simulink model "Autovessel_medPI"  (R2018a)
settings: Solver=FixedStepAuto  StartTime=0.0  StopTime=inf  RelTol=1e-3  EnableMultiTasking=on
libraries: arduinolib x4, simulink x2
settings Model: SimulationMode=external  ExtModeTrigDuration=2  Creator=Christoffer Lauknes  LastModifiedBy=Christoffer Lauknes
settings OptimizationCC: EnhancedBackFolding=on  PassReuseOutputArgsThreshold=0  MaxStackSize=64  OptimizeBlockOrder=speed  DifferentSizesBufferReuse=on  OptimizationCustomize=off
settings DebuggingCC: ParameterTunabilityLossMsg=error
settings HardwareCC: ProdBitPerInt=16  ProdBitPerPointer=16  ProdBitPerSizeT=16  ProdBitPerPtrDiffT=16  ProdLargestAtomicFloat=None  ProdWordSize=8  ProdHWDeviceType=Atmel->AVR  UseEmbeddedCoderFeatures=off
settings SFSimCC: MATLABDynamicMemAlloc=off
settings RTWCC: SystemTargetFile=ert.tlc  HardwareBoard=Arduino Mega 2560  TLCOptions=-aInlineSetEventsForThisBaseRateFcn=TLC_FALSE -aSuppressMultiTaskScheduler=TLC_FALSE -aRateBasedStepFcn=1  TemplateMakefile=ert_default_tmf  GenerateReport=on  Toolchain=Arduino AVR  BuildConfiguration=Faster Runs  LaunchReport=on
settings CodeAppCC: ForceParamTrailComments=on  OperatorAnnotations=on
settings ERTTargetCC: ERTCustomFileBanners=off  SupportContinuousTime=on  SupportNonInlinedSFcns=on  RemoveResetFunc=off  SupportVariableSizeSignals=on  ModelStepFunctionPrototypeControlCompliant=off

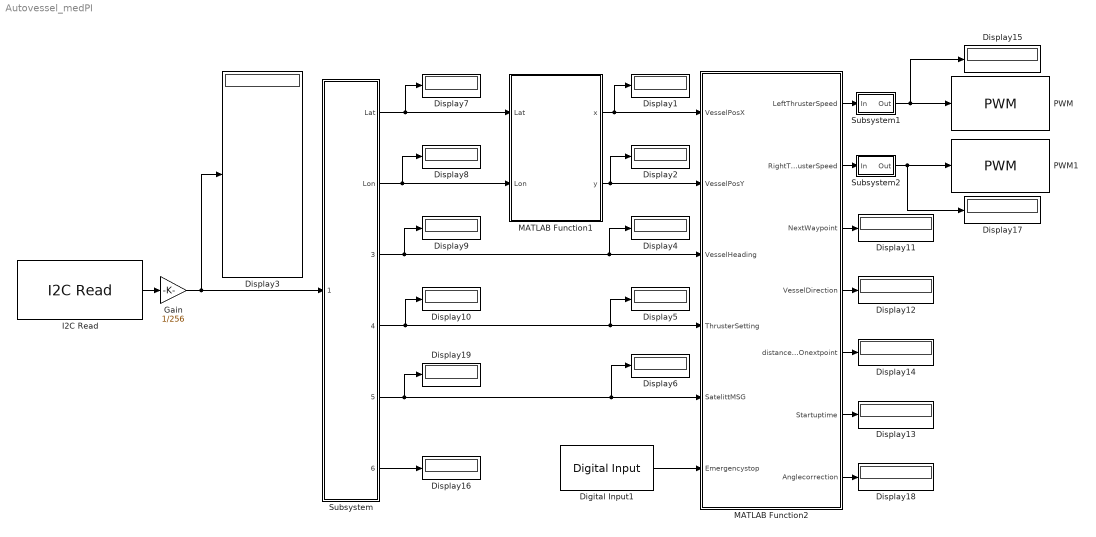
== system Autovessel_medPI ==
  Digital Input1 : arduinolib/Digital Input  pinNumber=30  sampleTime=0.1  blockPlatform=arduino
      settings: SourceProductName=Simulink Support Package for Arduino Hardware
  Display{1..19} (19 alike) : Display
  Gain : Gain  Gain=1/256  OutDataTypeStr=double
  I2C Read : arduinolib/I2C Read  SlaveAddress_=hex2dec( '48' )  RegisterAddressEnable=off  RegisterAddress_=hex2dec( '20' )  Datatype=uint16  ByteOrder=Big Endian  Datalength_=13  SampleTime_=0.1  blockPlatform=arduino
      settings: SourceProductName=Simulink Support Package for Arduino Hardware  SourceProductBaseCode=ARDUINO
  MATLAB Function1 : MATLAB Function  TreatAsAtomicUnit=on
  MATLAB Function2 : MATLAB Function  TreatAsAtomicUnit=on
  PWM : arduinolib/PWM  pinNumber=10  EnableInputFrequency=off  InitialFrequency=2000  InitialDutyCycle=0  NotificationType=None  blockPlatform=arduino
  PWM1 : arduinolib/PWM  pinNumber=12  EnableInputFrequency=off  InitialFrequency=2000  InitialDutyCycle=0  NotificationType=None  blockPlatform=arduino
  Subsystem : Subsystem
  Subsystem1 : Subsystem
  Subsystem2 : Subsystem
  wires:
  MATLAB Function2/1(LeftThrusterSpeed) -> Subsystem1/1(In)
  MATLAB Function2/2(RightThrusterSpeed) -> Subsystem2/1(In)
  MATLAB Function2/3(NextWaypoint) -> Display11/1
  Subsystem/6(Counter) -> Display16/1
  MATLAB Function2/5(distanceTOnextpoint) -> Display14/1
  Subsystem/3(Course) -> Display9/1, Display4/1, MATLAB Function2/3(VesselHeading)
  MATLAB Function2/4(VesselDirection) -> Display12/1
  Subsystem/4(Setting) -> Display10/1, Display5/1, MATLAB Function2/4(ThrusterSetting)
  Subsystem/2(Lon) -> Display8/1, MATLAB Function1/2(Lon)
  Gain/1 -> Display3/1, Subsystem/1(Slavedata)
  MATLAB Function1/1(x) -> Display1/1, MATLAB Function2/1(VesselPosX)
  Subsystem/1(Lat) -> Display7/1, MATLAB Function1/1(Lat)
  MATLAB Function2/6(Startuptime) -> Display13/1
  Subsystem/5(Satelitt) -> Display19/1, Display6/1, MATLAB Function2/5(SatelittMSG)
  MATLAB Function1/2(y) -> Display2/1, MATLAB Function2/2(VesselPosY)
  I2C Read/1 -> Gain/1
  Digital Input1/1 -> MATLAB Function2/6(Emergencystop)
  MATLAB Function2/7(Anglecorrection) -> Display18/1
  Subsystem2/1(Out) -> PWM1/1, Display17/1
  Subsystem1/1(Out) -> PWM/1, Display15/1

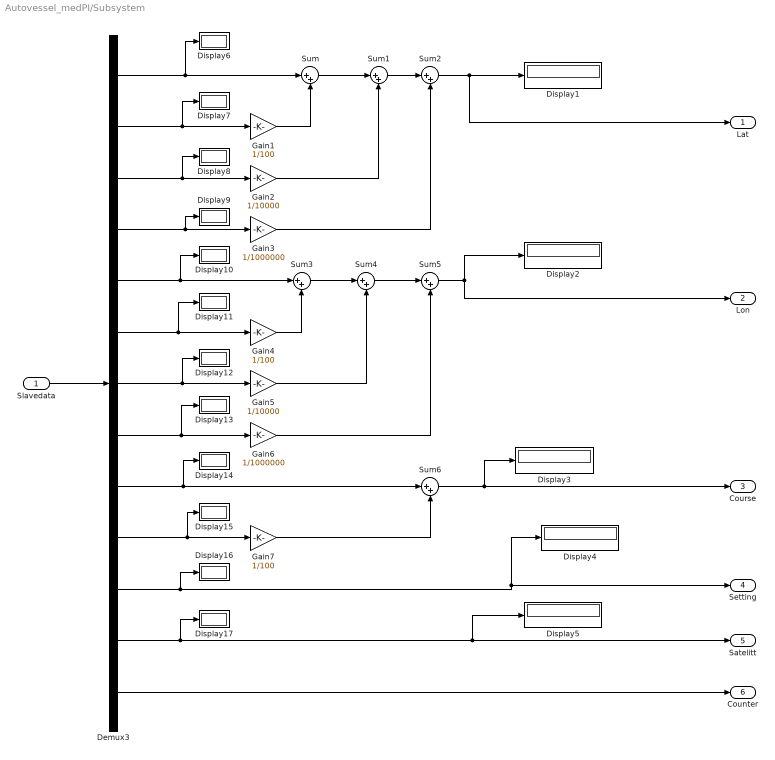
== system Autovessel_medPI/Subsystem ==
  Slavedata : Inport
  Demux3 : Demux  Outputs=13
  Display{1..17} (17 alike) : Display
      Display1 settings: Format=decimal (Stored Integer)
      Display2 settings: Format=decimal (Stored Integer)
      Display3 settings: Format=decimal (Stored Integer)
      Display4 settings: Format=decimal (Stored Integer)
      Display5 settings: Format=decimal (Stored Integer)
  Gain1 : Gain  Gain=1/100
  Gain2 : Gain  Gain=1/10000
  Gain3 : Gain  Gain=1/1000000
  Gain4 : Gain  Gain=1/100
  Gain5 : Gain  Gain=1/10000
  Gain6 : Gain  Gain=1/1000000
  Gain7 : Gain  Gain=1/100
  Sum{,1..6} (7 alike) : Sum  Inputs=|++
  Lat : Outport
  Lon : Outport  Port=2
  Course : Outport  Port=3
  Setting : Outport  Port=4
  Satelitt : Outport  Port=5
  Counter : Outport  Port=6
  wires:
  Sum6/1 -> Display3/1, Course/1
  Sum5/1 -> Display2/1, Lon/1
  Sum4/1 -> Sum5/1
  Sum3/1 -> Sum4/1
  Demux3/7 -> Display12/1, Gain5/1
  Sum/1 -> Sum1/1
  Slavedata/1 -> Demux3/1
  Gain7/1 -> Sum6/2
  Demux3/1 -> Display6/1, Sum/1
  Gain5/1 -> Sum4/2
  Demux3/2 -> Display7/1, Gain1/1
  Demux3/3 -> Gain2/1, Display8/1
  Sum2/1 -> Lat/1, Display1/1
  Demux3/5 -> Display10/1, Sum3/1
  Gain4/1 -> Sum3/2
  Gain1/1 -> Sum/2
  Demux3/4 -> Gain3/1, Display9/1
  Gain3/1 -> Sum2/2
  Demux3/8 -> Display13/1, Gain6/1
  Gain2/1 -> Sum1/2
  Gain6/1 -> Sum5/2
  Sum1/1 -> Sum2/1
  Demux3/10 -> Gain7/1, Display15/1
  Demux3/11 -> Display16/1, Setting/1, Display4/1
  Demux3/12 -> Display17/1, Satelitt/1, Display5/1
  Demux3/9 -> Display14/1, Sum6/1
  Demux3/6 -> Display11/1, Gain4/1
  Demux3/13 -> Counter/1

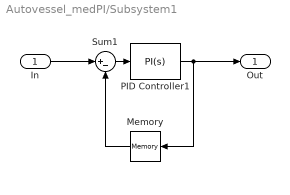
== system Autovessel_medPI/Subsystem1 ==
  In : Inport
  Memory : Memory  InheritSampleTime=on
  PID Controller1 : simulink/Continuous/PID Controller  Controller=PI  TimeDomain=Continuous-time  SampleTime=-1  IntegratorMethod=Forward Euler  FilterMethod=Forward Euler  Form=Parallel  UseFilter=on  ControllerParametersSource=internal  P=0.5  I=0.8  D=0  N=100  InitialConditionSource=internal  InitialConditionForIntegrator=0  InitialConditionForFilter=0  ExternalReset=none  LimitOutput=off  UpperSaturationLimit=inf  LowerSaturationLimit=-inf  LinearizeAsGain=on  AntiWindupMode=none  Kb=1  TrackingMode=off  Kt=1  PParamMin=[]  PParamMax=[]  IParamMin=[]  IParamMax=[]  DParamMin=[]  DParamMax=[]  NParamMin=[]  NParamMax=[]  KbParamMin=[]  KbParamMax=[]  KtParamMin=[]  KtParamMax=[]  POutMin=[]  POutMax=[]  IOutMin=[]  IOutMax=[]  DOutMin=[]  DOutMax=[]  NOutMin=[]  NOutMax=[]  KbOutMin=[]  KbOutMax=[]  KtOutMin=[]  KtOutMax=[]  IntegratorOutMin=[]  IntegratorOutMax=[]  FilterOutMin=[]  FilterOutMax=[]  SumOutMin=[]  SumOutMax=[]  SumI1OutMin=[]  SumI1OutMax=[]  SumI2OutMin=[]  SumI2OutMax=[]  SumI3OutMin=[]  SumI3OutMax=[]  SumDOutMin=[]  SumDOutMax=[]  SaturationOutMin=[]  SaturationOutMax=[]  IntegratorContinuousStateAttributes=''  IntegratorStateMustResolveToSignalObject=off  IntegratorRTWStateStorageClass=Auto  FilterContinuousStateAttributes=''  FilterStateMustResolveToSignalObject=off  FilterRTWStateStorageClass=Auto  DifferentiatorICPrevScaledInput=0  DifferentiatorOutMin=[]  DifferentiatorOutMax=[]  FilterDiffOutCoefMin=[]  FilterDiffOutCoefMax=[]  SumDenOutMin=[]  SumDenOutMax=[]  SumNumOutMin=[]  SumNumOutMax=[]  ReciprocalOutMin=[]  ReciprocalOutMax=[]  DivideOutMin=[]  DivideOutMax=[]  TunerSelectOption=Transfer Function Based (PID Tuner App)
  Sum1 : Sum  Inputs=|+-
  Out : Outport
  wires:
  In/1 -> Sum1/1
  PID Controller1/1 -> Memory/1, Out/1
  Sum1/1 -> PID Controller1/1
  Memory/1 -> Sum1/2

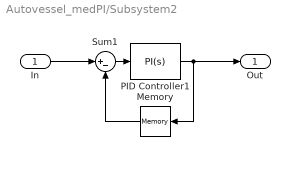
== system Autovessel_medPI/Subsystem2 ==
  In : Inport
  Memory : Memory  InheritSampleTime=on
  PID Controller1 : simulink/Continuous/PID Controller  Controller=PI  TimeDomain=Continuous-time  SampleTime=-1  IntegratorMethod=Forward Euler  FilterMethod=Forward Euler  Form=Parallel  UseFilter=on  ControllerParametersSource=internal  P=0.5  I=0.8  D=0  N=100  InitialConditionSource=internal  InitialConditionForIntegrator=0  InitialConditionForFilter=0  ExternalReset=none  LimitOutput=off  UpperSaturationLimit=inf  LowerSaturationLimit=-inf  LinearizeAsGain=on  AntiWindupMode=none  Kb=1  TrackingMode=off  Kt=1  PParamMin=[]  PParamMax=[]  IParamMin=[]  IParamMax=[]  DParamMin=[]  DParamMax=[]  NParamMin=[]  NParamMax=[]  KbParamMin=[]  KbParamMax=[]  KtParamMin=[]  KtParamMax=[]  POutMin=[]  POutMax=[]  IOutMin=[]  IOutMax=[]  DOutMin=[]  DOutMax=[]  NOutMin=[]  NOutMax=[]  KbOutMin=[]  KbOutMax=[]  KtOutMin=[]  KtOutMax=[]  IntegratorOutMin=[]  IntegratorOutMax=[]  FilterOutMin=[]  FilterOutMax=[]  SumOutMin=[]  SumOutMax=[]  SumI1OutMin=[]  SumI1OutMax=[]  SumI2OutMin=[]  SumI2OutMax=[]  SumI3OutMin=[]  SumI3OutMax=[]  SumDOutMin=[]  SumDOutMax=[]  SaturationOutMin=[]  SaturationOutMax=[]  IntegratorContinuousStateAttributes=''  IntegratorStateMustResolveToSignalObject=off  IntegratorRTWStateStorageClass=Auto  FilterContinuousStateAttributes=''  FilterStateMustResolveToSignalObject=off  FilterRTWStateStorageClass=Auto  DifferentiatorICPrevScaledInput=0  DifferentiatorOutMin=[]  DifferentiatorOutMax=[]  FilterDiffOutCoefMin=[]  FilterDiffOutCoefMax=[]  SumDenOutMin=[]  SumDenOutMax=[]  SumNumOutMin=[]  SumNumOutMax=[]  ReciprocalOutMin=[]  ReciprocalOutMax=[]  DivideOutMin=[]  DivideOutMax=[]  TunerSelectOption=Transfer Function Based (PID Tuner App)
  Sum1 : Sum  Inputs=|+-
  Out : Outport
  wires:
  In/1 -> Sum1/1
  PID Controller1/1 -> Memory/1, Out/1
  Sum1/1 -> PID Controller1/1
  Memory/1 -> Sum1/2

== matlab function Autovessel_medPI/MATLAB Function1 ==
  data: x output; Lat input; y output; Lon input
function  [x,y] = deg2utm(Lat,Lon)
% -------------------------------------------------------------------------
% [x,y,utmzone] = deg2utm(Lat,Lon)
%
% Description: Function to convert lat/lon vectors into UTM coordinates (WGS84).
% Some code has been extracted from UTM.m function by Gabriel Ruiz Martinez.
%
% Inputs:
%    Lat: Latitude vector.   Degrees.  +ddd.ddddd  WGS84
%    Lon: Longitude vector.  Degrees.  +ddd.ddddd  WGS84
%
% Outputs:
%    x, y , utmzone.   See example
%
% Example 1:
%    Lat=[40.3154333; 46.283900; 37.577833; 28.645650; 38.855550; 25.061783];
%    Lon=[-3.4857166; 7.8012333; -119.95525; -17.759533; -94.7990166; 121.640266];
%    [x,y,utmzone] = deg2utm(Lat,Lon);
%    fprintf('%7.0f ',x)
%       458731  407653  239027  230253  343898  362850
%    fprintf('%7.0f ',y)
%      4462881 5126290 4163083 3171843 4302285 2772478
%    utmzone =
%       30 T
%       32 T
%       11 S
%       28 R
%       15 S
%       51 R
%
% Example 2: If you have Lat/Lon coordinates in Degrees, Minutes and Seconds
%    LatDMS=[40 18 55.56; 46 17 2.04];
%    LonDMS=[-3 29  8.58;  7 48 4.44];
%    Lat=dms2deg(mat2dms(LatDMS)); %convert into degrees
%    Lon=dms2deg(mat2dms(LonDMS)); %convert into degrees
%    [x,y,utmzone] = deg2utm(Lat,Lon)
%
% Author: 
%   Rafael Palacios
%   Universidad Pontificia Comillas
%   Madrid, Spain
% Version: Apr/06, Jun/06, Aug/06, Aug/06
% Aug/06: fixed a problem (found by Rodolphe Dewarrat) related to southern 
%    hemisphere coordinates. 
% Aug/06: corrected m-Lint warnings
%-------------------------------------------------------------------------

% Argument checking
%
error(nargchk(2, 2, nargin));  %2 arguments required
n1=length(Lat);
n2=length(Lon);
if (n1~=n2)
   error('Lat and Lon vectors should have the same length');
end


% Memory pre-allocation
%
x=zeros(n1,1);
y=zeros(n1,1);
%utmzone(n1,:)='60 X';

% Main Loop
%
for i=1:n1
   la=Lat(i);
   lo=Lon(i);

   sa = 6378137.000000 ; sb = 6356752.314245;
         
   %e = ( ( ( sa ^ 2 ) - ( sb ^ 2 ) ) ^ 0.5 ) / sa;
   e2 = ( ( ( sa ^ 2 ) - ( sb ^ 2 ) ) ^ 0.5 ) / sb;
   e2cuadrada = e2 ^ 2;
   c = ( sa ^ 2 ) / sb;
   %alpha = ( sa - sb ) / sa;             %f
   %ablandamiento = 1 / alpha;   % 1/f

   lat = la * ( pi / 180 );
   lon = lo * ( pi / 180 );

   Huso = fix( ( lo / 6 ) + 31);
   S = ( ( Huso * 6 ) - 183 );
   deltaS = lon - ( S * ( pi / 180 ) );

   if (la<-72), Letra='C';
   elseif (la<-64), Letra='D';
   elseif (la<-56), Letra='E';
   elseif (la<-48), Letra='F';
   elseif (la<-40), Letra='G';
   elseif (la<-32), Letra='H';
   elseif (la<-24), Letra='J';
   elseif (la<-16), Letra='K';
   elseif (la<-8), Letra='L';
   elseif (la<0), Letra='M';
   elseif (la<8), Letra='N';
   elseif (la<16), Letra='P';
   elseif (la<24), Letra='Q';
   elseif (la<32), Letra='R';
   elseif (la<40), Letra='S';
   elseif (la<48), Letra='T';
   elseif (la<56), Letra='U';
   elseif (la<64), Letra='V';
   elseif (la<72), Letra='W';
   else Letra='X';
   end

   a = cos(lat) * sin(deltaS);
   epsilon = 0.5 * log( ( 1 +  a) / ( 1 - a ) );
   nu = atan( tan(lat) / cos(deltaS) ) - lat;
   v = ( c / ( ( 1 + ( e2cuadrada * ( cos(lat) ) ^ 2 ) ) ) ^ 0.5 ) * 0.9996;
   ta = ( e2cuadrada / 2 ) * epsilon ^ 2 * ( cos(lat) ) ^ 2;
   a1 = sin( 2 * lat );
   a2 = a1 * ( cos(lat) ) ^ 2;
   j2 = lat + ( a1 / 2 );
   j4 = ( ( 3 * j2 ) + a2 ) / 4;
   j6 = ( ( 5 * j4 ) + ( a2 * ( cos(lat) ) ^ 2) ) / 3;
   alfa = ( 3 / 4 ) * e2cuadrada;
   beta = ( 5 / 3 ) * alfa ^ 2;
   gama = ( 35 / 27 ) * alfa ^ 3;
   Bm = 0.9996 * c * ( lat - alfa * j2 + beta * j4 - gama * j6 );
   xx = epsilon * v * ( 1 + ( ta / 3 ) ) + 500000;
   yy = nu * v * ( 1 + ta ) + Bm;

   if (yy<0)
       yy=9999999+yy;
   end

   x(i)=xx;
   y(i)=yy;
end

== matlab function Autovessel_medPI/MATLAB Function2 ==
  data: LeftThrusterSpeed output; VesselPosX input; VesselPosY input; VesselHeading input; ThrusterSetting input; SatelittMSG input; RightThrusterSpeed output; Emergencystop input; NextWaypoint output; VesselDirection output; distanceTOnextpoint output; Startuptime output; Anglecorrection output
function [LeftThrusterSpeed, RightThrusterSpeed, NextWaypoint, VesselDirection, distanceTOnextpoint, Startuptime, Anglecorrection] = NavigationLOS(VesselPosX, VesselPosY, VesselHeading, ThrusterSetting, SatelittMSG, Emergencystop)

%% Parameters
%Rk=Cirkcle sorounding waypoints
%Rv = LOS circle surrounding the vessel
%X_k = X posision, next waypoint
%Y_k = Y posision, next waypoint
%X_k_1 = X posision, last waypoint
%Y_k_1 = Y posision, last waypoint
% delta_x = Distance between next and last waypoint, x dirrection
%delta_y = Distance between next and last waypoint, y dirrection
% i = determins waypoint
TurnConstantL = 3;
TurnConstantR = -3;
InitializationTime = 40;
VesselDirection = 0; 
Vh = 0;
leftThrusterRatio = 0;
rightThrusterRatio = 0;
LeftThrusterSpeed = 0;
RightThrusterSpeed = 0;
SpeedTObattery = 0;
delta_x = 0;
delta_y = 0;
NextWaypoint = 0;
YAWangle=0;
Anglecorrection = 0;

%Radius surroundg vessel and waypoints
Rv = 7;
Rk = 5;

persistent X_k_1;
if isempty(X_k_1)
    X_k_1 = VesselPosX;
end

persistent Y_k_1;
if isempty(Y_k_1)
    Y_k_1 = VesselPosY;
end

persistent i; 
if isempty(i) 
    i = 1;
end

persistent STOP;
if isempty (STOP)
    STOP = 0;
end

persistent StartupDelay;
if isempty(StartupDelay)
    StartupDelay = 0;
end
Startuptime = StartupDelay;

%Matrix with waypoint in UTM coordinates
GPS = [ 472808 6472535;
    472755 6472540;
    472757 6472501;
    472808 6472505;
    ];

posision = GPS;

%Sets hompeposision as next waypoint   
if SatelittMSG == 1
    i=7;
end


%% 
%Vessel posision, heading and speed
Xc = VesselPosX;
Yc = VesselPosY;
Vh = VesselHeading;
BatterySetting = ThrusterSetting;

%Correcting vesselcourse
if Vh <= pi/2
    YAWangle = 90*pi/180 - Vh;
elseif Vh > pi/2
    YAWangle = (360+90)*pi/180 - Vh;
end

%Waypoints
X_k = posision(i,1); %Next waypoint x
Y_k = posision(i,2); %Next waypoint y




%% Navigation
%Calculating LOS point
delta_x = X_k - X_k_1;
delta_y = Y_k - Y_k_1;

if( delta_x==0 )
    X_los = X_k_1;   % x_los = x_k;
    
    if( delta_y > 0 )
      Y_los = Yc + Rv;
    else                  % delta_y < 0
      Y_los = Yc - Rv;
    end
else % delta_x~=0
    d = delta_y/delta_x;
    e = X_k_1;
    f = Y_k_1;
    g = -d*e + f;
    a = 1 + d^2;
    b = 2*(d*g - d*Yc - Xc);
    c = Xc^2 + Yc^2 + g^2 - (Rv)^2 - 2*g*Yc;

    if ( delta_x > 0 )
      X_los = (-b + sqrt(b^2 - 4*a*c) )/(2*a);
    else % delta_x < 0
      X_los = (-b - sqrt(b^2 - 4*a*c) )/(2*a);
    end
    Y_los = d*(X_los - e) + f;
end

%Angle of the line between the vessel and the LOS point
LOSpointAngle = atan((Y_los - Yc)/(X_los-Xc));


if LOSpointAngle < 0
    LOSpointAngle = LOSpointAngle + 2*pi;
end

%Selects correct LOSpointAngle
if (Y_los - Yc) > 0 && pi < LOSpointAngle && LOSpointAngle < 2*pi
    LOSpointAngle = LOSpointAngle - pi;

elseif (Y_los - Yc) < 0 && 0 < LOSpointAngle && LOSpointAngle < pi
    LOSpointAngle = LOSpointAngle + pi;
end

%calculates difference between LOSpointAngle and YAWangle
%called corrAngle
corrAngle = (LOSpointAngle - YAWangle);

%Selects smallest corrAngle to achieve the right course
if corrAngle > pi
    corrAngle = corrAngle - 2*pi;
elseif corrAngle < -pi
    corrAngle = corrAngle + 2*pi;
end



%% Thruster control


 %Selcts ratio beween thruster to navigate towards LOS point
if corrAngle < 0
     leftThrusterRatio = 0;
     rightThrusterRatio = (corrAngle/(pi))*TurnConstantR;
elseif corrAngle > 0
     leftThrusterRatio = (corrAngle/(pi))*TurnConstantL;
     rightThrusterRatio = 0;
elseif corrAngle == 0
     leftThrusterRatio = 0;
     rightThrusterRatio = 0;  
end
    
    
%%prevent pwm signal above 187.5
    
if leftThrusterRatio < -1 
     leftThrusterRatio = -1;
elseif leftThrusterRatio > 1
     leftThrusterRatio = 1;
end

if rightThrusterRatio < -1
     rightThrusterRatio = -1;
elseif rightThrusterRatio > 1
     rightThrusterRatio = 1;
end


%Desired motorspeed based on battery level and power from solarpanel
%Emergency stop and arming of motorcontrollers
%Differance in PWM singal to the thruster to manuver the vessel
    
if Emergencystop == true && StartupDelay >= InitializationTime && STOP<1
     if (BatterySetting == 3)
      LeftThrusterSpeed =  147.5 + 40 * leftThrusterRatio;
      RightThrusterSpeed = 147.5 + 40 * rightThrusterRatio;
      
      elseif (BatterySetting == 2)
      LeftThrusterSpeed =  152.5 + 35 * leftThrusterRatio;
      RightThrusterSpeed = 152.5 + 35 * rightThrusterRatio;
      
      else 
      LeftThrusterSpeed =  157.5 + 30 * leftThrusterRatio;
      RightThrusterSpeed = 157.5 + 30 * rightThrusterRatio;
     end
     
     
%Vessel moving at the start to get vesseldirection from GPS     
      
elseif StartupDelay <= InitializationTime && Emergencystop == true && STOP<1
       LeftThrusterSpeed = 160;
       RightThrusterSpeed = 160;
       StartupDelay = StartupDelay + 1;
       pause(1);
      
      %Arming thrusters
else                     %Emergencystop == false
   LeftThrusterSpeed = 187.5;
   RightThrusterSpeed = 187.5;

 
end



%% Choosing next waypoint and setting past waypoint
distanceToWaypoint = sqrt((X_k-Xc)^2+(Y_k-Yc)^2);
if(distanceToWaypoint <= Rk)
   X_k_1 = X_k;
   Y_k_1 = Y_k;
   i = i+1;

%Restarts matrix when last point is reached or stops boat when homeposision 
%is reached
   if (i==4)
     i = 1;
   elseif (i==5)
     STOP=1;
   end

end


%% Outputs for monitoring during testing on land
NextWaypoint = i;
VesselDirection = VesselHeading*180/pi;
distanceTOnextpoint = distanceToWaypoint;
Anglecorrection = corrAngle*180/pi;



end
